simulink model "updated_quad"  (R2017a)
settings: Solver=VariableStepAuto  StartTime=0.0  StopTime=500  RelTol=1e-3  EnableMultiTasking=on
undefined symbols (not defined in the file or in its folder): magnitude
libraries: mpclib x1
settings Model: Creator=sherief nabeeh  LastModifiedBy=sherief nabeeh
settings OptimizationCC: LifeSpan=inf
settings DebuggingCC: SFUnexpectedBacktrackingDiag=warning  SFNoUnconditionalDefaultTransitionDiag=warning  SFExecutionAtInitializationDiag=none
settings GRTTargetCC: TargetLangStandard=C89/C90 (ANSI)  GeneratePreprocessorConditionals=Disable all
settings ConfigComp: CovMetricSettings=dw  CovHtmlReporting=on  CovSaveCumulativeToWorkspaceVar=on  CovSaveSingleToWorkspaceVar=on  CovExternalEMLEnable=off

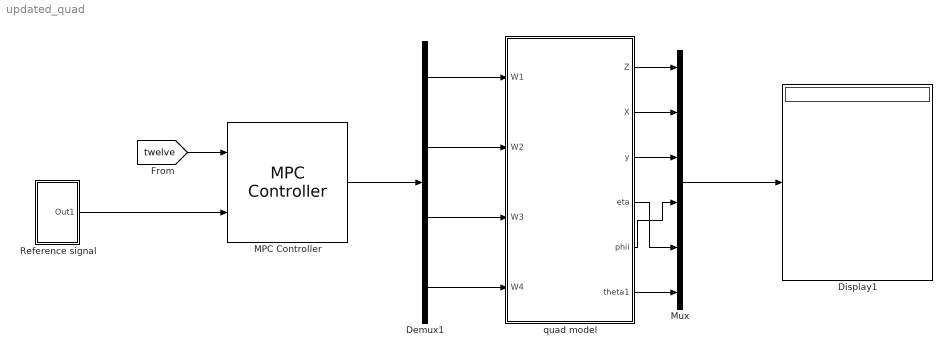
== system updated_quad ==
  Demux1 : Demux
  Display1 : Display
  MPC Controller : mpclib/MPC Controller  SCDEnableBlockLinearizationSpecification=on  mpcobj=mpcobj  is_multiple=0  enable_value=0  return_u0=off  ref_from_ws=off  ref_signal_name=[]  ref_preview=off  md_from_ws=off  md_signal_name=[]  md_preview=off  from_project=off  project_file=MPCtask.mat  md_inport=off  mv_inport=off  cost_outport=off  return_sequence=off  return_qpstatus=off  return_state=off  state_inport=off  lims_inport=off  ywt_inport=off  is_designfromscratch=0  uwt_inport=off  duwt_inport=off  rhoeps_inport=off  uref_inport=off  n_ts=0.04  n_mv=4  n_md=0  n_ud=0  n_mo=12  n_uo=0  BlockDataType=double  SampleTimeInherited=off  switch_inport=off
  Mux : Mux  Inputs=6
  Reference signal : Subsystem
  quad model : Subsystem
  wires:
  MPC Controller/1 -> Demux1/1
  [twelve] -> MPC Controller/1
  Reference signal/1(Out1) -> MPC Controller/2
  Mux/1 -> Display1/1
  quad model/1(Z) -> Mux/1
  quad model/2(X) -> Mux/2
  quad model/3(y) -> Mux/3
  quad model/5(phii) -> Mux/4
  quad model/4(eta) -> Mux/5
  quad model/6(theta1) -> Mux/6
  Demux1/1 -> quad model/1(W1)
  Demux1/2 -> quad model/2(W2)
  Demux1/3 -> quad model/3(W3)
  Demux1/4 -> quad model/4(W4)

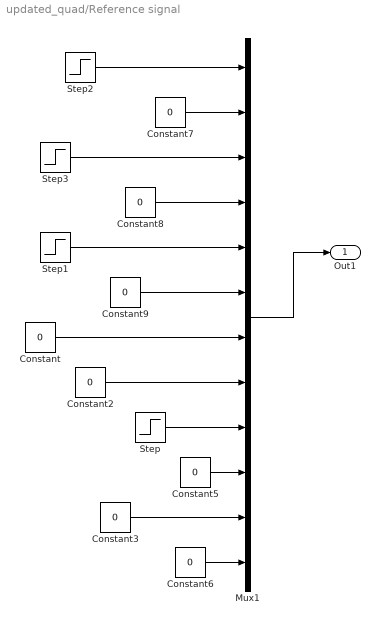
== system updated_quad/Reference signal ==
  Constant{,2..3,5..9} (8 alike) : Constant  Value=0
  Mux1 : Mux  Inputs=12
  Step : Step  After=5  SampleTime=0
  Step1 : Step  Time=10  After=-5  SampleTime=0
  Step2 : Step  Time=10  After=50  SampleTime=0
  Step3 : Step  Time=0  After=0  SampleTime=0
  Out1 : Outport
  wires:
  Step2/1 -> Mux1/1
  Constant7/1 -> Mux1/2
  Constant8/1 -> Mux1/4
  Constant9/1 -> Mux1/6
  Step3/1 -> Mux1/3
  Step1/1 -> Mux1/5
  Mux1/1 -> Out1/1
  Constant/1 -> Mux1/7
  Constant2/1 -> Mux1/8
  Step/1 -> Mux1/9
  Constant6/1 -> Mux1/12
  Constant3/1 -> Mux1/11
  Constant5/1 -> Mux1/10

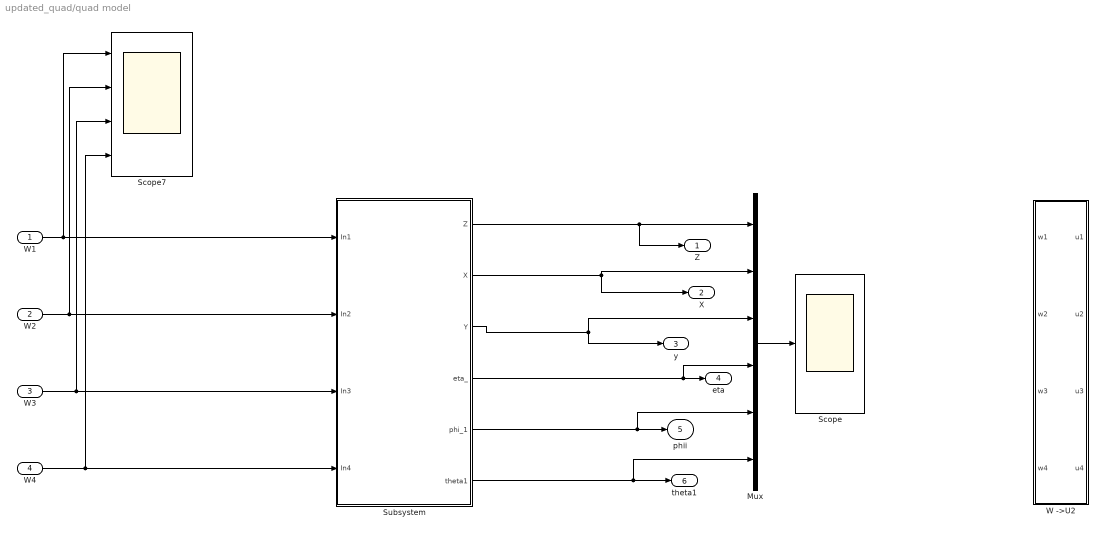
== system updated_quad/quad model ==
  W1 : Inport
  W2 : Inport  Port=2
  W3 : Inport  Port=3
  W4 : Inport  Port=4
  Mux : Mux  Inputs=6
  Scope : Scope
  Scope7 : Scope  NumInputPorts=4
  Subsystem : Subsystem
  W ->U2 : Subsystem
  Z : Outport
  X : Outport  Port=2
  y : Outport  Port=3
  eta : Outport  Port=4
  phii : Outport  Port=5
  theta1 : Outport  Port=6
  wires:
  Subsystem/1(Z) -> Z/1, Mux/1
  Subsystem/3(Y) -> Mux/3, y/1
  Subsystem/5(phi_1) -> Mux/5, phii/1
  Subsystem/6(theta1) -> Mux/6, theta1/1
  Subsystem/4(eta_) -> Mux/4, eta/1
  Subsystem/2(X) -> Mux/2, X/1
  Mux/1 -> Scope/1
  W2/1 -> Subsystem/2(In2), Scope7/2
  W3/1 -> Subsystem/3(In3), Scope7/3
  W4/1 -> Subsystem/4(In4), Scope7/4
  W1/1 -> Subsystem/1(In1), Scope7/1

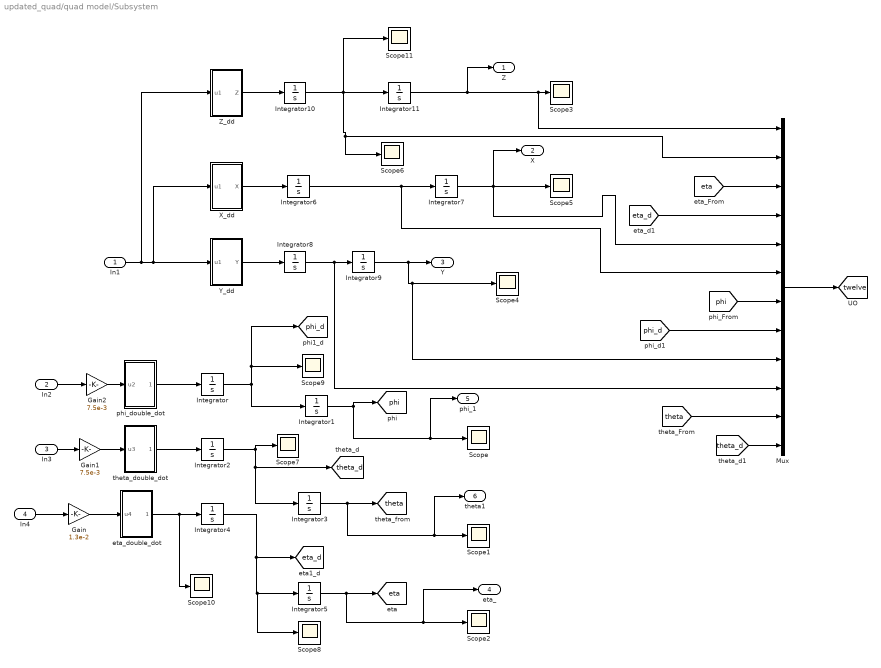
== system updated_quad/quad model/Subsystem ==
  In1 : Inport
  In2 : Inport  Port=2
  In3 : Inport  Port=3
  In4 : Inport  Port=4
  Gain : Gain  Gain=1.3e-2
  Gain1 : Gain  Gain=7.5e-3
  Gain2 : Gain  Gain=7.5e-3
  Integrator{,1..11} (12 alike) : Integrator
  Mux : Mux  Inputs=12
  Scope{,1..11} (12 alike) : Scope
  "X_dd " : Subsystem
  Y_dd : Subsystem
  Z_dd : Subsystem
  eta_double_dot : Subsystem
  phi_double_dot : Subsystem
  theta_double_dot : Subsystem
  Z : Outport
  X : Outport  Port=2
  Y : Outport  Port=3
  eta_ : Outport  Port=4
  phi_1 : Outport  Port=5
  theta1 : Outport  Port=6
  tag scope: eta=global, eta_d=global, phi=global, phi_d=global, theta=global, theta_d=global, twelve=global
  wires:
  Integrator11/1 -> Z/1, Mux/1, Scope3/1
  eta_double_dot/1(phi_1) -> Scope10/1, Integrator4/1
  In4/1 -> Gain/1
  Integrator6/1 -> Mux/6, Integrator7/1
  Integrator7/1 -> Mux/5, X/1, Scope5/1
  Integrator2/1 -> Integrator3/1, [theta_d], Scope7/1
  Integrator/1 -> Scope9/1, [phi_d], Integrator1/1
  phi_double_dot/1(phi_) -> Integrator/1
  In2/1 -> Gain2/1
  Integrator4/1 -> Scope8/1, Integrator5/1, [eta_d]
  Integrator1/1 -> [phi], phi_1/1, Scope/1
  "X_dd "/1(X) -> Integrator6/1
  Y_dd/1(Y) -> Integrator8/1
  In3/1 -> Gain1/1
  Integrator9/1 -> Y/1, Mux/9, Scope4/1
  In1/1 -> Y_dd/1(u1), "X_dd "/1(u1), Z_dd/1(u1)
  Z_dd/1(Z) -> Integrator10/1
  Integrator3/1 -> theta1/1, Scope1/1, [theta]
  Integrator5/1 -> eta_/1, Scope2/1, [eta]
  theta_double_dot/1(phi_1) -> Integrator2/1
  Mux/1 -> [twelve]
  Integrator10/1 -> Scope11/1, Mux/2, Scope6/1, Integrator11/1
  [eta] -> Mux/3
  [eta_d] -> Mux/4
  [phi] -> Mux/7
  [phi_d] -> Mux/8
  Integrator8/1 -> Mux/10, Integrator9/1
  [theta] -> Mux/11
  [theta_d] -> Mux/12
  Gain/1 -> eta_double_dot/1(u4)
  Gain1/1 -> theta_double_dot/1(u3)
  Gain2/1 -> phi_double_dot/1(u2)

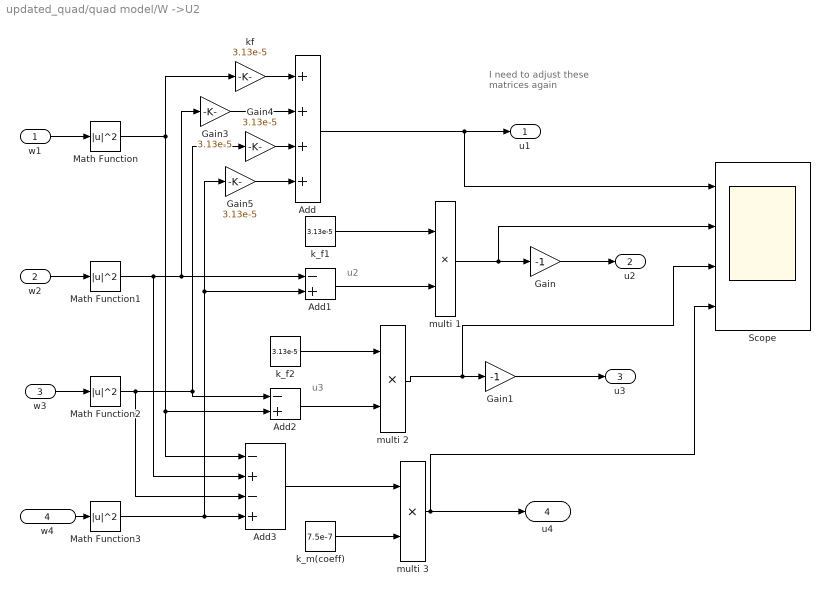
== system updated_quad/quad model/W ->U2 ==
  note: I need to adjust these matrices again
  note: u2
  note: u3
  w1 : Inport
  w2 : Inport  Port=2
  w3 : Inport  Port=3
  w4 : Inport  Port=4
  Add : Sum  Inputs=++++
  Add1 : Sum  Inputs=-+
  Add2 : Sum  Inputs=-+
  Add3 : Sum  Inputs=-+-+
  Gain : Gain  Gain=-1
  Gain1 : Gain  Gain=-1
  Gain3 : Gain  Gain=3.13e-5
  Gain4 : Gain  Gain=3.13e-5
  Gain5 : Gain  Gain=3.13e-5
  Math Function{,1..3} (4 alike) : Math  Operator=magnitude^2  SaturateOnIntegerOverflow=on
  Scope : Scope  NumInputPorts=4
  k_f1 : Constant  Value=3.13e-5
  k_f2 : Constant  Value=3.13e-5
  k_m(coeff) : Constant  Value=7.5e-7
  kf : Gain  Gain=3.13e-5
  multi 1 : Product  Inputs=**
  multi 2 : Product  Inputs=**
  multi 3 : Product  Inputs=**
  u1 : Outport
  "u2 " : Outport  Port=2
  u3 : Outport  Port=3
  u4 : Outport  Port=4
  wires:
  Add/1 -> u1/1, Scope/1
  multi 3/1 -> Scope/4, u4/1
  k_f2/1 -> multi 2/1
  Add2/1 -> multi 2/2
  multi 2/1 -> Scope/3, Gain1/1
  Add3/1 -> multi 3/1
  Math Function2/1 -> Add3/3, Add2/1, Gain4/1
  Math Function1/1 -> Add3/2, Add1/1, Gain3/1
  Math Function3/1 -> Add1/2, Gain5/1, Add3/4
  multi 1/1 -> Scope/2, Gain/1
  k_m(coeff)/1 -> multi 3/2
  Math Function/1 -> Add3/1, Add2/2, kf/1
  k_f1/1 -> multi 1/1
  Add1/1 -> multi 1/2
  kf/1 -> Add/1
  Gain3/1 -> Add/2
  Gain4/1 -> Add/3
  Gain5/1 -> Add/4
  w4/1 -> Math Function3/1
  w3/1 -> Math Function2/1
  w2/1 -> Math Function1/1
  w1/1 -> Math Function/1
  Gain/1 -> "u2 "/1
  Gain1/1 -> u3/1

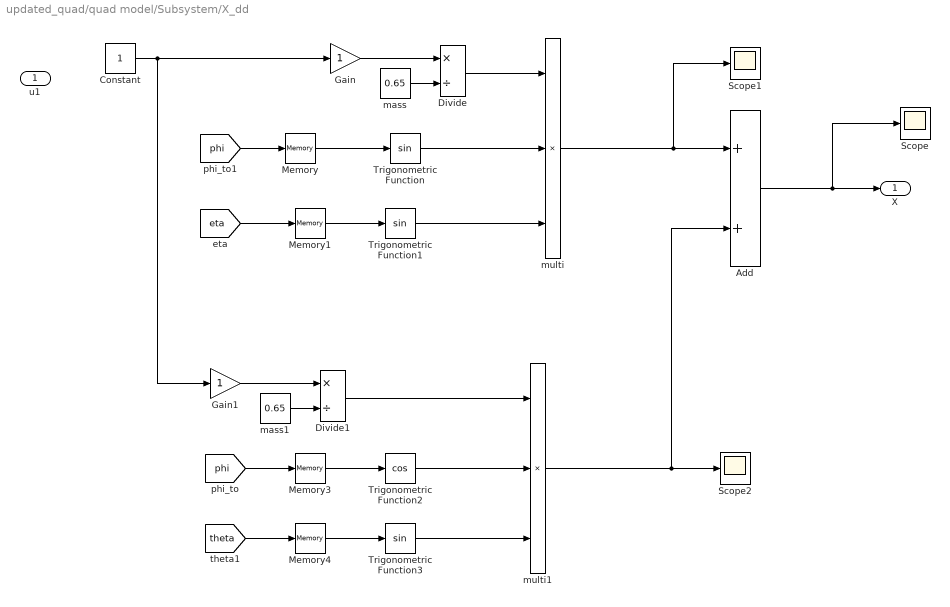
== system updated_quad/quad model/Subsystem/X_dd  ==
  u1 : Inport
  Add : Sum
  Constant : Constant
  Divide : Product  Inputs=*/
  Divide1 : Product  Inputs=*/
  Gain : Gain
  Gain1 : Gain
  Memory{,1,3..4} (4 alike) : Memory
  Scope : Scope
  Scope1 : Scope
  Scope2 : Scope
  Trigonometric Function : Trigonometry
  Trigonometric Function1 : Trigonometry
  Trigonometric Function2 : Trigonometry  Operator=cos
  Trigonometric Function3 : Trigonometry
  mass : Constant  Value=0.65
  mass1 : Constant  Value=0.65
  multi : Product  Inputs=***
  multi1 : Product  Inputs=***
  X : Outport
  wires:
  multi/1 -> Scope1/1, Add/1
  Add/1 -> Scope/1, X/1
  mass/1 -> Divide/2
  Gain/1 -> Divide/1
  [phi] -> Memory/1
  [eta] -> Memory1/1
  multi1/1 -> Scope2/1, Add/2
  [theta] -> Memory4/1
  [phi] -> Memory3/1
  Trigonometric Function2/1 -> multi1/2
  Trigonometric Function3/1 -> multi1/3
  Divide/1 -> multi/1
  Trigonometric Function/1 -> multi/2
  Trigonometric Function1/1 -> multi/3
  Memory/1 -> Trigonometric Function/1
  Memory1/1 -> Trigonometric Function1/1
  Memory3/1 -> Trigonometric Function2/1
  Memory4/1 -> Trigonometric Function3/1
  mass1/1 -> Divide1/2
  Gain1/1 -> Divide1/1
  Divide1/1 -> multi1/1
  Constant/1 -> Gain1/1, Gain/1

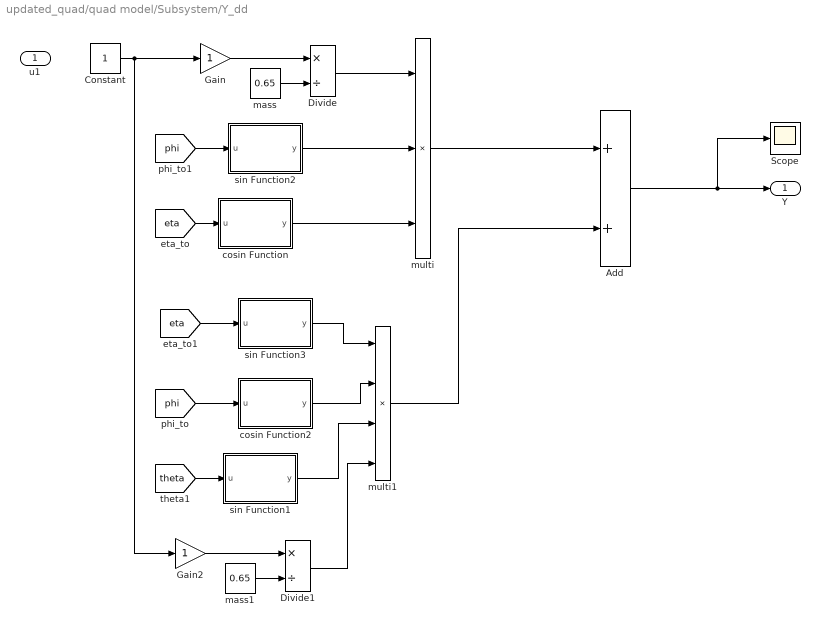
== system updated_quad/quad model/Subsystem/Y_dd ==
  u1 : Inport
  Add : Sum
  Constant : Constant
  Divide : Product  Inputs=*/
  Divide1 : Product  Inputs=*/
  Gain : Gain
  Gain2 : Gain
  Scope : Scope
  cosin Function : MATLAB Function  TreatAsAtomicUnit=on
  cosin Function2 : MATLAB Function  TreatAsAtomicUnit=on
  mass : Constant  Value=0.65
  mass1 : Constant  Value=0.65
  multi : Product  Inputs=***
  multi1 : Product  Inputs=****
  sin Function1 : MATLAB Function  TreatAsAtomicUnit=on
  sin Function2 : MATLAB Function  TreatAsAtomicUnit=on
  sin Function3 : MATLAB Function  TreatAsAtomicUnit=on
  Y : Outport
  wires:
  multi/1 -> Add/1
  Add/1 -> Scope/1, Y/1
  mass/1 -> Divide/2
  Gain/1 -> Divide/1
  [eta] -> cosin Function/1(u)
  multi1/1 -> Add/2
  [theta] -> sin Function1/1(u)
  [eta] -> sin Function3/1(u)
  [phi] -> cosin Function2/1(u)
  cosin Function2/1(y) -> multi1/2
  sin Function3/1(y) -> multi1/1
  sin Function1/1(y) -> multi1/3
  Divide/1 -> multi/1
  cosin Function/1(y) -> multi/3
  sin Function2/1(y) -> multi/2
  [phi] -> sin Function2/1(u)
  mass1/1 -> Divide1/2
  Gain2/1 -> Divide1/1
  Divide1/1 -> multi1/4
  Constant/1 -> Gain2/1, Gain/1

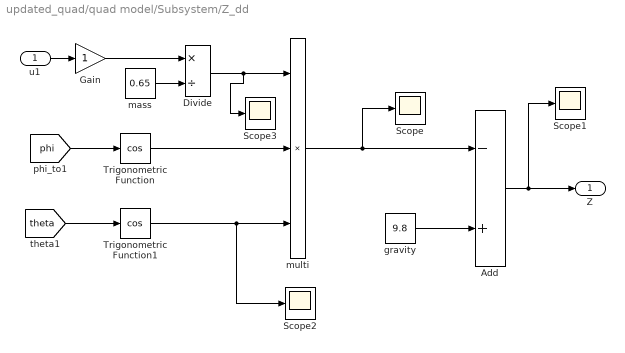
== system updated_quad/quad model/Subsystem/Z_dd ==
  u1 : Inport
  Add : Sum  Inputs=-+
  Divide : Product  Inputs=*/
  Gain : Gain
  Scope{,1..3} (4 alike) : Scope
  Trigonometric Function : Trigonometry  Operator=cos
  Trigonometric Function1 : Trigonometry  Operator=cos
  gravity : Constant  Value=9.8
  mass : Constant  Value=0.65
  multi : Product  Inputs=***
  Z : Outport
  wires:
  u1/1 -> Gain/1
  multi/1 -> Scope/1, Add/1
  Add/1 -> Scope1/1, Z/1
  mass/1 -> Divide/2
  Gain/1 -> Divide/1
  [theta] -> Trigonometric Function1/1
  gravity/1 -> Add/2
  Trigonometric Function1/1 -> Scope2/1, multi/3
  Trigonometric Function/1 -> multi/2
  [phi] -> Trigonometric Function/1
  Divide/1 -> Scope3/1, multi/1

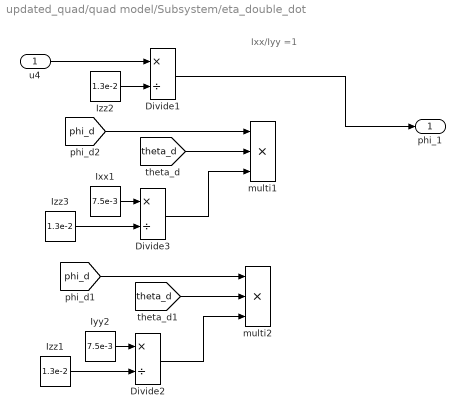
== system updated_quad/quad model/Subsystem/eta_double_dot ==
  note: Ixx/Iyy =1
  u4 : Inport
  Divide1 : Product  Inputs=*/
  Divide2 : Product  Inputs=*/
  Divide3 : Product  Inputs=*/
  Ixx1 : Constant  Value=7.5e-3
  Iyy2 : Constant  Value=7.5e-3
  Izz1 : Constant  Value=1.3e-2
  Izz2 : Constant  Value=1.3e-2
  Izz3 : Constant  Value=1.3e-2
  multi1 : Product  Inputs=***
  multi2 : Product  Inputs=***
  phi_1 : Outport
  wires:
  u4/1 -> Divide1/1
  Divide1/1 -> phi_1/1
  Izz2/1 -> Divide1/2
  Divide2/1 -> multi2/3
  [phi_d] -> multi2/1
  [theta_d] -> multi2/2
  Divide3/1 -> multi1/3
  Izz3/1 -> Divide3/2
  Ixx1/1 -> Divide3/1
  [phi_d] -> multi1/1
  [theta_d] -> multi1/2
  Izz1/1 -> Divide2/2
  Iyy2/1 -> Divide2/1

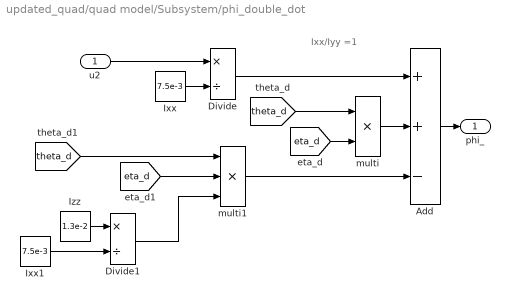
== system updated_quad/quad model/Subsystem/phi_double_dot ==
  note: Ixx/Iyy =1
  u2 : Inport
  Add : Sum  Inputs=++-
  Divide : Product  Inputs=*/
  Divide1 : Product  Inputs=*/
  Ixx : Constant  Value=7.5e-3
  Ixx1 : Constant  Value=7.5e-3
  Izz : Constant  Value=1.3e-2
  multi : Product  Inputs=**
  multi1 : Product  Inputs=***
  phi_ : Outport
  wires:
  Divide/1 -> Add/1
  u2/1 -> Divide/1
  multi/1 -> Add/2
  Add/1 -> phi_/1
  [theta_d] -> multi/1
  Ixx/1 -> Divide/2
  [eta_d] -> multi/2
  multi1/1 -> Add/3
  Divide1/1 -> multi1/3
  Ixx1/1 -> Divide1/2
  Izz/1 -> Divide1/1
  [theta_d] -> multi1/1
  [eta_d] -> multi1/2

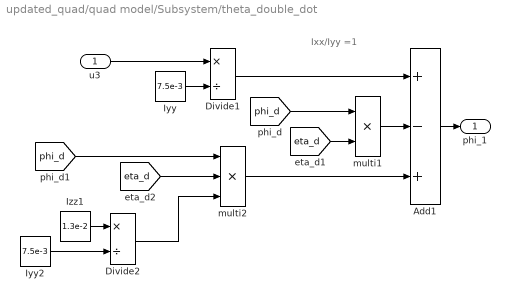
== system updated_quad/quad model/Subsystem/theta_double_dot ==
  note: Ixx/Iyy =1
  u3 : Inport
  Add1 : Sum  Inputs=+-+
  Divide1 : Product  Inputs=*/
  Divide2 : Product  Inputs=*/
  Iyy : Constant  Value=7.5e-3
  Iyy2 : Constant  Value=7.5e-3
  Izz1 : Constant  Value=1.3e-2
  multi1 : Product  Inputs=**
  multi2 : Product  Inputs=***
  phi_1 : Outport
  wires:
  Divide1/1 -> Add1/1
  u3/1 -> Divide1/1
  multi1/1 -> Add1/2
  Add1/1 -> phi_1/1
  [phi_d] -> multi1/1
  Iyy/1 -> Divide1/2
  [eta_d] -> multi1/2
  multi2/1 -> Add1/3
  Divide2/1 -> multi2/3
  Iyy2/1 -> Divide2/2
  Izz1/1 -> Divide2/1
  [phi_d] -> multi2/1
  [eta_d] -> multi2/2

== matlab function updated_quad/quad model/Subsystem/Y_dd/cosin Function ==
  data: u input; y output
function y = fcn(u)
%#codegen

y = cos(u);

== matlab function updated_quad/quad model/Subsystem/Y_dd/sin Function2 ==
  data: u input; y output
function y = fcn(u)
%#codegen

y = sin(u);

== matlab function updated_quad/quad model/Subsystem/Y_dd/sin Function1 ==
  data: u input; y output
function y = fcn(u)
%#codegen

y = sin(u);

== matlab function updated_quad/quad model/Subsystem/Y_dd/sin Function3 ==
  data: u input; y output
function y = fcn(u)
%#codegen

y = sin(u);

== matlab function updated_quad/quad model/Subsystem/Y_dd/cosin Function2 ==
  data: u input; y output
function y = fcn(u)
%#codegen

y = cos(u);
